simulink model "Missile"  (R2024a)
settings: Solver=ode45  StartTime=0.0  StopTime=80.0  RelTol=1e-3
values from neighbouring files (symbols this model uses):
  A = [-1.064 1; 290.26 0]    [missile.m]
  B = [-0.25 ; -331.40]    [missile.m]
  C = [-123.34 0; 0 1]    [missile.m]
  D = [-13.51; 0]    [missile.m]
  dT1 = 0.75    [missile.m]
  dT2 = 0.25    [missile.m]
  ELEV_INIT = 10000    [missile.m]
  ELEV_TARGET = 795    [missile.m]
  LAT_INIT = 34.2329    [missile.m]
  LAT_OBS = 34.61916    [missile.m]
  LAT_TARGET = 34.6588    [missile.m]
  LON_INIT = -119.4753    [missile.m]
  LON_OBS = -118.769745    [missile.m]
  LON_TARGET = -118.8429    [missile.m]
undefined symbols (not defined in the file or in its folder): Earth, K, L, WGS84
libraries: simulink x3, aerolibtransform2 x1, slpidlib x1, aerolibanimutils x1
settings Model: Creator=macbookair  LastModifiedBy=macbookair

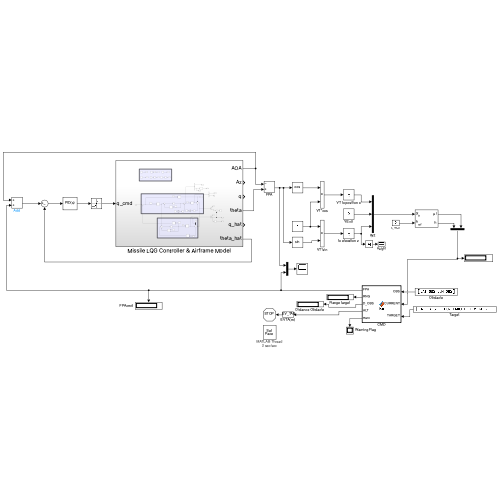
[thumbnail: Simulink's stored preview of the top-level diagram]
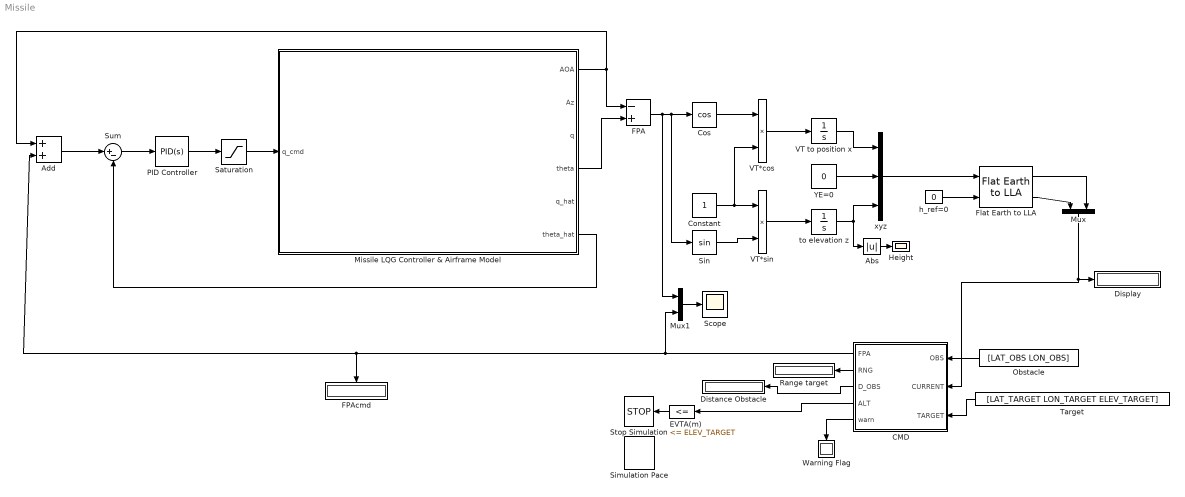
== system Missile ==
  Abs : Abs  SaturateOnIntegerOverflow=off
  Add : Sum
  CMD : MATLAB Function  TreatAsAtomicUnit=on
  Constant : Constant
  Cos : Trigonometry  Operator=cos
  Display : Display
  Distance Obstacle : Display
  "EVTA(m) " : simulink/Logic and Bit Operations/Compare To Constant  relop=<=  const=ELEV_TARGET  OutDataTypeStr=boolean
  FPA : Sum  Inputs=-+
  FPAcmd : Display
  Flat Earth to LLA : aerolibtransform2/Flat Earth to LLA  units=Metric (MKS)  ptype=Earth (WGS84)  F=1/298.257223563  R=6378137  refPosPort=off  LL0=[LAT_INIT LON_INIT]  psi=yaw_init
  Height : Scope
  Missile LQG Controller & Airframe Model : Subsystem
  Mux : Mux  Inputs=2
  Mux1 : Mux  Inputs=2
  Obstacle : Constant  Value=[LAT_OBS LON_OBS]
  PID Controller : slpidlib/PID Controller  Controller=PID  Form=Parallel  TimeDomain=Continuous-time  UseExternalTs=off  SampleTime=-1  IntegratorMethod=Forward Euler  FilterMethod=Forward Euler  ControllerParametersSource=internal  P=-1  I=0  UseKiTs=off  D=0  UseExternalDerivativeSource=off  N=100  UseFilter=on  TunerSelectOption=Transfer Function Based (PID Tuner App)  InitialConditionSource=internal  InitialConditionForIntegrator=0  InitialConditionForFilter=0  DifferentiatorICPrevScaledInput=0  ExternalReset=none  TrackingMode=off  Kt=1  LimitOutput=off  SatLimitsSource=internal  UpperSaturationLimit=inf  LowerSaturationLimit=-inf  LinearizeAsGain=on  AntiWindupMode=none  Kb=1  LimitIntegrator=off  UpperIntegratorSaturationLimit=inf  LowerIntegratorSaturationLimit=-inf  POutMin=[]  POutMax=[]  IOutMin=[]  IOutMax=[]  DOutMin=[]  DOutMax=[]  NOutMin=[]  NOutMax=[]  SumOutMin=[]  SumOutMax=[]  SaturationOutMin=[]  SaturationOutMax=[]  PParamMin=[]  PParamMax=[]  IParamMin=[]  IParamMax=[]  DParamMin=[]  DParamMax=[]  NParamMin=[]  NParamMax=[]  KbParamMin=[]  KbParamMax=[]  KtParamMin=[]  KtParamMax=[]  KbOutMin=[]  KbOutMax=[]  KtOutMin=[]  KtOutMax=[]  IntegratorOutMin=[]  IntegratorOutMax=[]  FilterOutMin=[]  FilterOutMax=[]  SumI1OutMin=[]  SumI1OutMax=[]  SumI2OutMin=[]  SumI2OutMax=[]  SumI3OutMin=[]  SumI3OutMax=[]  SumI4OutMin=[]  SumI4OutMax=[]  SumDOutMin=[]  SumDOutMax=[]  DifferentiatorOutMin=[]  DifferentiatorOutMax=[]  FilterDiffOutCoefMin=[]  FilterDiffOutCoefMax=[]  ReciprocalOutMin=[]  ReciprocalOutMax=[]  SumDenOutMin=[]  SumDenOutMax=[]  SumNumOutMin=[]  SumNumOutMax=[]  DivideOutMin=[]  DivideOutMax=[]  UdiffTsProdOutMin=[]  UdiffTsProdOutMax=[]  NTsProdOutMin=[]  NTsProdOutMax=[]  UintegralTsProdOutMin=[]  UintegralTsProdOutMax=[]  UngainTsProdOutMin=[]  UngainTsProdOutMax=[]  ClampingZeroOutDataTypeStr=Inherit: Inherit via back propagation  ClampingZeroOutMin=[]  ClampingZeroOutMax=[]  FilterDenConstantOutDataTypeStr=Inherit: Inherit via back propagation  FilterDenConstantOutMin=[]  FilterDenConstantOutMax=[]  PCopyOutDataTypeStr=Inherit: Inherit via back propagation  PCopyOutMin=[]  PCopyOutMax=[]  NCopyOutDataTypeStr=Inherit: Inherit via back propagation  NCopyOutMin=[]  NCopyOutMax=[]  IntegratorContinuousStateAttributes=''  IntegratorStateMustResolveToSignalObject=off  IntegratorRTWStateStorageClass=Auto  FilterContinuousStateAttributes=''  FilterStateMustResolveToSignalObject=off  FilterRTWStateStorageClass=Auto  ParallelPVariant=InternalParameters  IdealPVariant=Disabled  IVariant=InternalParameters  DVariant=InternalParameters  IntegratorVariant=Continuous  SatVariant=Disabled  AWVariant=Passthrough  PCopyVariant=Disabled  TRVariant=Disabled  FdbkBlocksVariant=Forward  IdealPFdbkVariant=Disabled  SatFdbkVariant=Disabled  DerivativeFilterVariant=ContFilter  NVariant=InternalParameters  NCopyVariant=Disabled  FilterICVariant=InternalICsFilter  IntegratorICVariant=InternalICs  ExternalResetVariant=Disabled  TRSumVariant=Passthrough  SumFdbkVariant=Disabled  SumVariant=Sum_PID  TsampFilterVariant=InternalTs  TsampNgainVariant=Passthrough  TsampIntegralVariant=Disabled_SignalSpec  ExternalSaturationOutDataTypeStr=Inherit: Same as second input  DerivativeSourceVariant=ErrorSignal
  Range target : Display
  Saturation : Saturate
  Scope : Scope
  Simulation Pace : aerolibanimutils/Simulation Pace  SimulationPace=2  SleepMode=MATLAB Thread  OutputPaceError=off  SampleTime=1/30
  Sin : Trigonometry
  Stop Simulation : Stop
  Sum : Sum  Inputs=|+-
  Target : Constant  Value=[LAT_TARGET LON_TARGET ELEV_TARGET]
  VT to position x : Integrator
  VT*cos : Product
  VT*sin : Product
  Warning Flag : Display
  YE=0 : Constant  Value=0
  h_ref=0 : Constant  Value=0
  to elevation z : Integrator  InitialCondition=-ELEV_INIT
  xyz : Mux  Inputs=3
  wires:
  to elevation z/1 -> Abs/1, xyz/3
  VT to position x/1 -> xyz/1
  VT*sin/1 -> to elevation z/1
  YE=0/1 -> xyz/2
  VT*cos/1 -> VT to position x/1
  Missile LQG Controller & Airframe Model/6(theta_hat) -> Sum/2
  Sin/1 -> VT*sin/2
  Cos/1 -> VT*cos/1
  Saturation/1 -> Missile LQG Controller & Airframe Model/1(q_cmd)
  Missile LQG Controller & Airframe Model/1(AOA) -> FPA/1, Add/1
  Add/1 -> Sum/1
  Constant/1 -> VT*sin/1, VT*cos/2
  FPA/1 -> Mux1/1, Sin/1, Cos/1
  PID Controller/1 -> Saturation/1
  Missile LQG Controller & Airframe Model/4(theta) -> FPA/2
  Sum/1 -> PID Controller/1
  Abs/1 -> Height/1
  xyz/1 -> Flat Earth to LLA/1
  h_ref=0/1 -> Flat Earth to LLA/2
  Flat Earth to LLA/1 -> Mux/2
  Flat Earth to LLA/2 -> Mux/1
  Target/1 -> CMD/3(TARGET)
  Obstacle/1 -> CMD/1(OBS)
  Mux/1 -> Display/1, CMD/2(CURRENT)
  CMD/2(RNG) -> Range target/1
  CMD/3(D_OBS) -> Distance Obstacle/1
  CMD/5(warn) -> Warning Flag/1
  CMD/1(FPA) -> Mux1/2, FPAcmd/1, Add/2
  Mux1/1 -> Scope/1
  CMD/4(ALT) -> "EVTA(m) "/1
  "EVTA(m) "/1 -> Stop Simulation/1

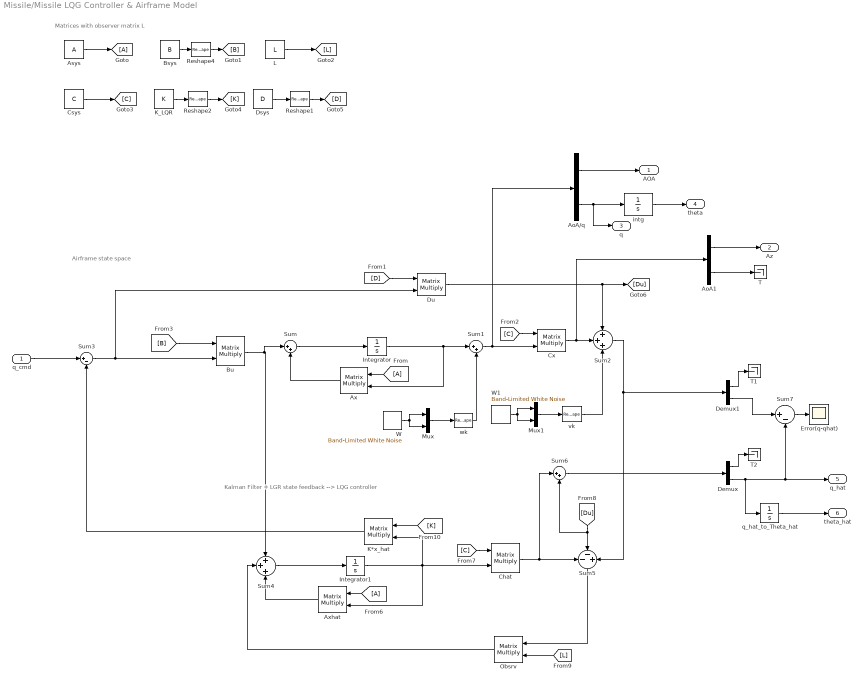
== system Missile/Missile LQG Controller & Airframe Model ==
  note: Airframe state space
  note: Kalman Filter + LGR state feedback --> LQG controller
  note: Matrices with observer matrix L
  q_cmd : Inport
  AoA/q : Demux  Outputs=2
  AoA1 : Demux  Outputs=2
  Asys : Constant  Value=A
  Ax : Product  Multiplication=Matrix(*)
  Axhat : Product  Multiplication=Matrix(*)
  Bsys : Constant  Value=B
  Bu : Product  Multiplication=Matrix(*)
  Chat : Product  Multiplication=Matrix(*)
  Csys : Constant  Value=C
  Cx : Product  Multiplication=Matrix(*)
  Demux : Demux  Outputs=2
  Demux1 : Demux  Outputs=2
  Dsys : Constant  Value=D
  Du : Product  Multiplication=Matrix(*)
  Error(q-qhat) : Scope
  From : From
  From6 : From
  Goto : Goto
  Integrator : Integrator
  Integrator1 : Integrator
  K*x_hat : Product  Multiplication=Matrix(*)
  K_LQR : Constant  Value=K
  L : Constant  Value=L
  Mux : Mux  Inputs=2
  Mux1 : Mux  Inputs=2
  Obsrv : Product  Multiplication=Matrix(*)
  Reshape1 : Reshape  OutputDimensionality=Customize  OutputDimensions=[2,1]
  Reshape2 : Reshape  OutputDimensionality=Customize  OutputDimensions=[1,2]
  Reshape4 : Reshape  OutputDimensionality=Customize  OutputDimensions=[2,1]
  Sum : Sum  Inputs=|++
  Sum1 : Sum  Inputs=|++
  Sum2 : Sum  Inputs=+++
  Sum3 : Sum  Inputs=|+-
  Sum4 : Sum  Inputs=+++
  Sum5 : Sum  Inputs=--+
  Sum6 : Sum  Inputs=|++
  Sum7 : Sum  Inputs=|+-
  T : Terminator
  T1 : Terminator
  T2 : Terminator
  W : simulink/Sources/Band-Limited White Noise  Cov=[0.0000001]  Ts=dT1  seed=[23341]
  W1 : simulink/Sources/Band-Limited White Noise  Cov=[0.00001]  Ts=dT2  seed=[23341]
  intg : Integrator
  q_hat_to_Theta_hat : Integrator
  vk : Reshape  OutputDimensionality=Customize  OutputDimensions=[2,1]
  wk : Reshape  OutputDimensionality=Customize  OutputDimensions=[2,1]
  AOA : Outport
  Az : Outport  Port=2
  q : Outport  Port=3
  theta : Outport  Port=4
  q_hat : Outport  Port=5
  theta_hat : Outport  Port=6
  wires:
  Sum4/1 -> Integrator1/1
  [L] -> Obsrv/2
  Sum5/1 -> Obsrv/1
  From6/1 -> Axhat/1
  [C] -> Cx/1
  Obsrv/1 -> Sum4/2
  W1/1 -> Mux1/1, Mux1/2
  wk/1 -> Sum1/2
  [C] -> Chat/1
  Reshape1/1 -> [D]
  [K] -> K*x_hat/1
  L/1 -> [L]
  Bsys/1 -> Reshape4/1
  Axhat/1 -> Sum4/3
  Sum6/1 -> Demux/1
  Ax/1 -> Sum/2
  q_hat_to_Theta_hat/1 -> theta_hat/1
  AoA/q/2 -> q/1, intg/1
  [B] -> Bu/1
  AoA/q/1 -> AOA/1
  Csys/1 -> [C]
  K*x_hat/1 -> Sum3/2
  Integrator/1 -> Ax/2, Sum1/1
  q_cmd/1 -> Sum3/1
  Mux/1 -> wk/1
  AoA1/2 -> T/1
  Chat/1 -> Sum6/1, Sum5/1
  From/1 -> Ax/1
  Asys/1 -> Goto/1
  Demux/1 -> T2/1
  Mux1/1 -> vk/1
  K_LQR/1 -> Reshape2/1
  Sum/1 -> Integrator/1
  Demux1/2 -> Sum7/1
  W/1 -> Mux/1, Mux/2
  vk/1 -> Sum2/3
  Dsys/1 -> Reshape1/1
  AoA1/1 -> Az/1
  Demux/2 -> q_hat/1, Sum7/2, q_hat_to_Theta_hat/1
  Sum7/1 -> Error(q-qhat)/1
  Sum3/1 -> Du/2, Bu/2
  Demux1/1 -> T1/1
  Bu/1 -> Sum/1, Sum4/1
  Reshape4/1 -> [B]
  Cx/1 -> AoA1/1, Sum2/2
  Sum1/1 -> AoA/q/1, Cx/2
  [D] -> Du/1
  [Du] -> Sum6/2, Sum5/2
  Du/1 -> Sum2/1, [Du]
  Sum2/1 -> Demux1/1, Sum5/3
  Integrator1/1 -> K*x_hat/2, Chat/2, Axhat/2
  Reshape2/1 -> [K]
  intg/1 -> theta/1

== matlab function Missile/CMD ==
  data: OBS input; FPA output; CURRENT input; TARGET input; RNG output; D_OBS output; ALT output; warn output
function [FPA,RNG,D_OBS,ALT,warn] = fcn(OBS, CURRENT, TARGET)

R = 6.371e3;
d2r = pi/180;

%OBSTACLE LOCATION
LAT_OBS = OBS(1);
LON_OBS = OBS(2);

%OBSTACLE THRESHOLD (ZONE)
thres = 2000; % 2km

%TARGET LOCATION
LAT_TARGET = TARGET(1);
LON_TARGET = TARGET(2);
ELEV_TARGET = TARGET(3);

%Current LOCATION
ELEV_CUR = CURRENT(1);
LAT_CUR = CURRENT(2);
LON_CUR = CURRENT(3);

%% distance to target
l1 = LAT_CUR*d2r;
u1 = LON_CUR*d2r;
l2 = LAT_TARGET*d2r;
u2 = LON_TARGET*d2r;
dh = abs(ELEV_TARGET-ELEV_CUR);

dl = l2-l1;
du = u2-u1;

a = sin(dl/2)^2+cos(l1)*cos(l2)*sin(du/2)^2;
c = 2 * atan2(sqrt(a),sqrt(1-a));
d = R*c; % horizontal distance (in m)

%% Distance from the obstacle
l3 = LAT_OBS * d2r;
u3 = LON_OBS * d2r;
dl = l3-l1;
du = u3-u1;

a = sin(dl/2)^2+cos(l1)*cos(l2)*sin(du/2)^2;
c = 2 * atan2(sqrt(a),sqrt(1-a));
d_obs = R*c; % horizontal distance (in m)


%% current range (from target) - range > distance
range = sqrt(d^2 + dh^2);

%% calculate commanded flight path setpoint based on d_obs, range
if abs(d_obs)>=thres
    w = 0;
    FPA_CMD = atan(dh/d);
else
    % when in the obstacle zone warning flag
    w = 1;
    FPA_CMD = 0;
end

FPA = FPA_CMD;
RNG = range;
D_OBS = d_obs;
warn = w;
ALT = ELEV_CUR;
